simulink model "AirRefueling_Platform_Varyingmass"  (R2023a)
settings: Solver=VariableStepAuto  StartTime=0.0  StopTime=100  FixedStep=0.01  RelTol=1e-3  EnableMultiTasking=on
InitFcn:
  | F16_Init
values from neighbouring files (symbols this model uses):
  A_define = A(1:12,1:12)    [F16_Init.m]
  airSpeed = 393.72    [F16_Init.m]
  alpha0 = trimAlpha*180/pi    (= 6.62393794015)    [F16_Init.m]
  altitude = 9843    [F16_Init.m]
  B_define = A(1:12,13:16)    [F16_Init.m]
  b_ref = 30.0    (= 30)    [F16_Init.m]
  C = [ 1,0,0,zeros(1,15) ... (first row only)    [F16_Init.m]
  C2m = [C(1,:) ... (first row only)    [F16_Init.m]
  C_la = [1,0,zeros(1,4)]    [F16_Init.m]
  C_lon = [1,0,zeros(1,4);0,1,zeros(1,4)]    [F16_Init.m]
  Cdr_ = 0.8    [HoseDrogue_Parameter.m]
  d_f_rc = [3.75;0;-1.75]    [F16_Init.m]
  d_pr_cam = d_pr_rc - d_cam_rc    [F16_Init.m]
  d_pr_rc = [7.6;0.50;-2.44]    [F16_Init.m]
  dLEF = 0    [F16_Init.m]
  dtheta10 = zeros(1,N)    [HoseDrogue_Parameter.m]
  dtheta20 = zeros(1,N)    [HoseDrogue_Parameter.m]
  fi_flag = 1    [F16_Init.m]
  height = 3000    [HoseDrogue_Parameter.m]
  Inertia = [9496,0,-982.0;0,55814.0,0;-982.0,0,63100.0]    [F16_Init.m]
  k_reel = 0.5    [HoseDrogue_Parameter.m]
  Kc = [ ... (first row only)    [F16_Init.m]
  kd = 500    [HoseDrogue_Parameter.m]
  Ki = zeros(4,3)    [F16_Init.m]
  Ki_la = -k_la(:,9)    [F16_Init.m]
  Ki_lon = -k_lon(:,9:10)    [F16_Init.m]
  Kp = zeros(4,18)    [F16_Init.m]
  kp_la = Kp_define(3:4,[2,4,6,9,10,12])    [F16_Init.m]
  kp_lon = Kp_define(1:2,[1,3,5,7,8,11])    [F16_Init.m]
  l0 = (length-l1)/(N-1)    (= 1.44444444444)    [HoseDrogue_Parameter.m]
  l1 = 2    [HoseDrogue_Parameter.m]
  l_density = 4.1    [HoseDrogue_Parameter.m]
  m0 = l0*l_density    (= 5.92222222222)    [HoseDrogue_Parameter.m]
  mass = 636.94    [F16_Init.m]
  Mdr = 29.5    [HoseDrogue_Parameter.m]
  N = 10    [HoseDrogue_Parameter.m]    (also in bsp3.m)
  p0_rc = [-30;1;8]    [F16_Init.m]
  Rdr = 0.305    [HoseDrogue_Parameter.m]
  Rl = 0.0336    [HoseDrogue_Parameter.m]
  T_reel_initial = 1610    [HoseDrogue_Parameter.m]
  theta10 = theta1_100    [HoseDrogue_Parameter.m]
  theta20 = theta2_100    [HoseDrogue_Parameter.m]
  trim_ail = 0.00874607850103852    (= 0.00874607850104)    [F16_Init.m]
  trim_control = [trim_thrust;trim_ele;trim_ail;trim_rud]    [F16_Init.m]
  trim_ele = -2.97973164860638    (= -2.97973164861)    [F16_Init.m]
  trim_rud = 0.0680302158182712    (= 0.0680302158183)    [F16_Init.m]
  trim_state = [0;0;0;0;trimAlpha;0;airSpeed;trimAlpha;0;0;0;0]    [F16_Init.m]
  trim_state1 = [trim_state;0;0;0;0;0;0]    [F16_Init.m]
  trim_thrust = 2279.08519954656    (= 2279.08519955)    [F16_Init.m]
  visual_err = [0.07;0.04;-1.21]    [F16_Init.m]
  vt0 = [120;0;0]    [HoseDrogue_Parameter.m]
undefined symbols (not defined in the file or in its folder): A_la_define, A_lon_define, B_la_define, B_lon_define, CC_la, CC_lon, dockingPoint, F, Light, MIL, STD, v_oil
libraries: aerolibconvert2 x13, etargetslib x11, dspnetwork x10, aerolibasang x8, aerolibatmos2 x3, aerolibobsolete x3, simulink x2, aerolibwind2 x2, aerolibadyn x2, sharedtransform x2, aerolibutil x2, vrlib x1
(part 2 of 4)

== system AirRefueling_Platform_Varyingmass/Receiver system/Controller ==
  note: u
  note: -kx
  note: u'
  note: e
  note: 跟踪控制
      | 设计反馈矩阵 Ki 使得误差 e 收敛为0
  note: x'=Ax+Bu
      | 增稳控制 u = Kp * x
      | 设计反馈矩阵 Kp 配置极点
  Ori_states : Inport
  C : Gain  Commented=on  Gain=C  Multiplication=Matrix(K*u) (u vector)
  Constant : Constant  Commented=on  Value=trim_control
  Demux : Demux  Commented=on
  Demux1 : Demux  Commented=on  Outputs=3
  Display : Display  Commented=on
  Gain : Gain  Commented=on  Gain=1000
  Gain1 : Gain  Commented=on  Gain=[1,0,0;0,0,-1;0,1,0]  Multiplication=Matrix(K*u) (u vector)
  Integrator : Integrator  Commented=on
  Integrator1 : Integrator  Commented=on
  Integrator2 : Integrator  Commented=on
  Ki : Gain  Commented=on  Gain=Ki  Multiplication=Matrix(K*u) (u vector)
  Kp : Gain  Commented=on  Gain=Kp  Multiplication=Matrix(K*u) (u vector)
  Length Conversion : aerolibconvert2/Length Conversion  Commented=on  IU=m  OU=ft
  Mux : Mux  Commented=on
  Mux3 : Mux  Commented=on  Inputs=3
  Observer1 : Subsystem
  Saturation : Saturate  Commented=on  UpperLimit=15  LowerLimit=-15
  Sum : Sum  Commented=on  Inputs=|++
  Sum2 : Sum  Commented=on  Inputs=|+-
  Sum3 : Sum  Commented=on  Inputs=+|-
  Sum4 : Sum  Inputs=|++
  pri_sys_controller1 : Subsystem
  sec_sys_controller1 : Subsystem
  Out1 : Outport
  wires:
  Sum2/1 -> Demux1/1
  C/1 -> Sum2/2
  Mux3/1 -> Ki/1
  Demux1/2 -> Integrator1/1
  Integrator1/1 -> Mux3/2
  Integrator/1 -> Mux3/1
  Demux1/3 -> Integrator2/1
  Integrator2/1 -> Mux3/3
  Length Conversion/1 -> Sum2/1
  Demux1/1 -> Saturation/1
  Ki/1 -> Sum3/1
  Kp/1 -> Sum3/2
  Sum3/1 -> Demux/1
  Saturation/1 -> Integrator/1
  Demux/2 -> Mux/2
  Demux/3 -> Mux/3
  Demux/4 -> Mux/4
  Demux/1 -> Gain/1
  Gain/1 -> Mux/1
  ? -> Gain1/1
  Gain1/1 -> Length Conversion/1
  Constant/1 -> Sum/2
  Mux/1 -> Sum/1
  sec_sys_controller1/1(Sec_inputs) -> Observer1/1(Sec_input), Sum4/2
  Ori_states/1 -> Observer1/2(Ori_states)
  Sum4/1 -> Out1/1
  Observer1/1(Sec_Obv_States) -> sec_sys_controller1/2(Sec_Obv_States)
  Observer1/2(Pri_Obv_States) -> sec_sys_controller1/1(Pri_Obv_States), pri_sys_controller1/1(Pri_Obv_States)
  pri_sys_controller1/1(Pri_inputs) -> Sum4/1

== system AirRefueling_Platform_Varyingmass/Receiver system/F16 Nonlinear Model ==
  u2 : Inport
  u4 : Inport  Port=2
  Variable Mass Model : Subsystem
  constant mass model : Subsystem
  state2 : Outport
  Out2 : Outport  Port=2
  state3 : Outport  Port=3
  wires:
  u4/1 -> Variable Mass Model/1(u4)
  Variable Mass Model/1(state2) -> state2/1
  Variable Mass Model/2(Out2) -> Out2/1
  Variable Mass Model/3(state3) -> state3/1
  u2/1 -> constant mass model/1(u2)
  constant mass model/1(V_wind) -> Variable Mass Model/2(Wind Velocity)
  constant mass model/2(W_wind) -> Variable Mass Model/3(Wind Angular Rates)

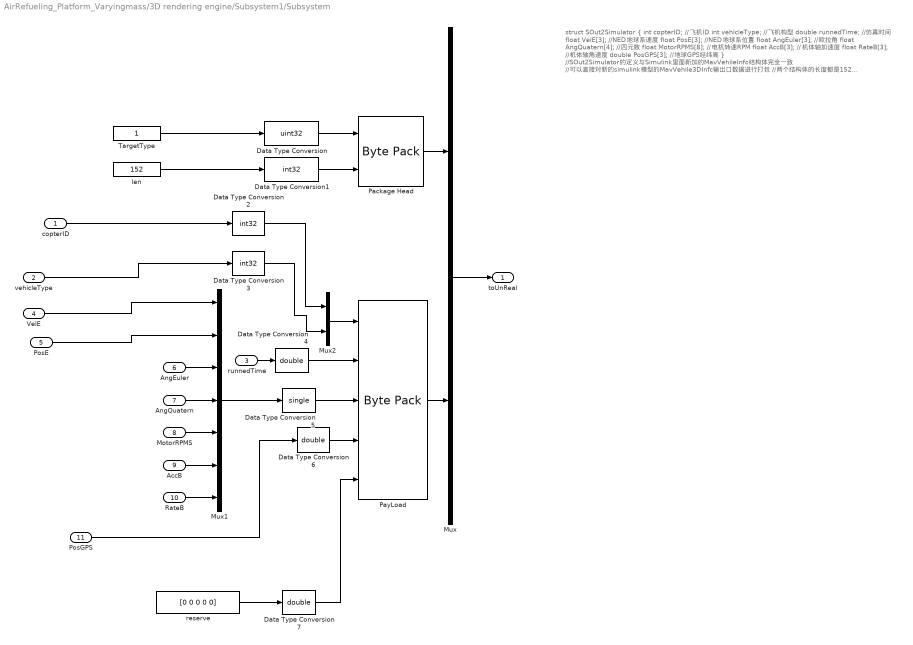
== system AirRefueling_Platform_Varyingmass/3D rendering engine/Subsystem1/Subsystem ==
  note: struct SOut2Simulator
      | {
      | int copterID; //飞机ID
      | int vehicleType; //飞机构型
      | double runnedTime; //仿真时间
      | float VelE[3]; //NED地球系速度
      | float PosE[3]; //NED地球系位置
      | float AngEuler[3]; //欧拉角
      | float AngQuatern[4]; //四元数
      | float MotorRPMS[8]; //电机转速RPM
      | float AccB[3]; //机体轴加速度
      | float RateB[3]; //机体轴角速度
      | double PosGPS[3]; //地球GPS经纬高
      | }
      |
      | //SOut2Simulator的定义与Simulink里面新加的MavVehileInfo结构体完全一致
      | //可以直接对新的simulink模型的MavVehile3DInfo输出口数据进行打包
      | //两个结构体的长度都是152
      | sizeof(SOut2Simulator) = sizeof(MavVehileInfo) = 152
      |
      | 打包封装的结构体为
      | typedef struct _netDataShort
      | {
      | TargetType tg; //这里目前随便填，写1即可 uint32
      | int len; //这个长度为传输结构体长度，目前是152
      | char payload[192]; //这里面前152位存放了SOut2Simulator结构体数据，后面的40位保留
      | }netDataShort;
      |
      | //UDP包的总长度为200
      | sizeof(netDataShort) = 200
      |
      | //发送的UDP端口号为：20010
  copterID : Inport  PortDimensions=1
  vehicleType : Inport  Port=2  PortDimensions=1
  runnedTime : Inport  Port=3  PortDimensions=1
  "VelE " : Inport  Port=4  PortDimensions=3
  PosE : Inport  Port=5  PortDimensions=3
  AngEuler : Inport  Port=6  PortDimensions=3
  AngQuatern : Inport  Port=7  PortDimensions=4
  MotorRPMS : Inport  Port=8  PortDimensions=8
  AccB : Inport  Port=9  PortDimensions=3
  RateB : Inport  Port=10  PortDimensions=3
  PosGPS : Inport  Port=11  PortDimensions=3
  Data Type Conversion : DataTypeConversion  OutDataTypeStr=uint32  SaturateOnIntegerOverflow=off  RndMeth=Floor
  Data Type Conversion1 : DataTypeConversion  OutDataTypeStr=int32  SaturateOnIntegerOverflow=off  RndMeth=Floor
  Data Type Conversion2 : DataTypeConversion  OutDataTypeStr=int32  SaturateOnIntegerOverflow=off  RndMeth=Floor
  Data Type Conversion3 : DataTypeConversion  OutDataTypeStr=int32  SaturateOnIntegerOverflow=off  RndMeth=Floor
  Data Type Conversion4 : DataTypeConversion  OutDataTypeStr=double  SaturateOnIntegerOverflow=off  RndMeth=Floor
  Data Type Conversion5 : DataTypeConversion  OutDataTypeStr=single  SaturateOnIntegerOverflow=off  RndMeth=Floor
  Data Type Conversion6 : DataTypeConversion  OutDataTypeStr=double  SaturateOnIntegerOverflow=off  RndMeth=Floor
  Data Type Conversion7 : DataTypeConversion  OutDataTypeStr=double  SaturateOnIntegerOverflow=off  RndMeth=Floor
  Mux : Mux  Inputs=2
  Mux1 : Mux  Inputs=7
  Mux2 : Mux  Inputs=2
  Package Head : etargetslib/Byte Pack  datatypes={'uint32','int32'}  byteAlign=4
  PayLoad : etargetslib/Byte Pack  datatypes={'int32','double','single','double','double'}  byteAlign=8
  TargetType : Constant  OutDataTypeStr=Inherit: Inherit via back propagation
  len : Constant  Value=152  OutDataTypeStr=Inherit: Inherit via back propagation
  reserve : Constant  Value=[0 0 0 0 0]  OutDataTypeStr=double
  toUnReal : Outport  VectorParamsAs1DForOutWhenUnconnected=off
  wires:
  runnedTime/1 -> Data Type Conversion4/1
  RateB/1 -> Mux1/7
  PayLoad/1 -> Mux/2
  "VelE "/1 -> Mux1/1
  Mux1/1 -> Data Type Conversion5/1
  PosGPS/1 -> Data Type Conversion6/1
  Package Head/1 -> Mux/1
  AccB/1 -> Mux1/6
  Mux/1 -> toUnReal/1
  MotorRPMS/1 -> Mux1/5
  AngQuatern/1 -> Mux1/4
  copterID/1 -> Data Type Conversion2/1
  len/1 -> Data Type Conversion1/1
  vehicleType/1 -> Data Type Conversion3/1
  PosE/1 -> Mux1/2
  TargetType/1 -> Data Type Conversion/1
  reserve/1 -> Data Type Conversion7/1
  Mux2/1 -> PayLoad/1
  AngEuler/1 -> Mux1/3
  Data Type Conversion5/1 -> PayLoad/3
  Data Type Conversion2/1 -> Mux2/1
  Data Type Conversion1/1 -> Package Head/2
  Data Type Conversion6/1 -> PayLoad/4
  Data Type Conversion/1 -> Package Head/1
  Data Type Conversion3/1 -> Mux2/2
  Data Type Conversion4/1 -> PayLoad/2
  Data Type Conversion7/1 -> PayLoad/5

== system AirRefueling_Platform_Varyingmass/Hose-drogue system/DRdynamics/HDU ==
  note: 第一根管子的a
  t_hose : Inport
  Compare To Zero : simulink/Logic and Bit Operations/Compare To Zero  Commented=on  relop=<=  OutDataTypeStr=boolean
  Divide : Product  Inputs=*/
  Integrator : Integrator  ExternalReset=rising  UpperSaturationLimit=0.3  LowerSaturationLimit=-0.3
  Integrator1 : Integrator  ExternalReset=rising  InitialCondition=l1
  MATLAB Function1 : MATLAB Function  TreatAsAtomicUnit=on
  MATLAB Function2 : MATLAB Function  TreatAsAtomicUnit=on
  Memory2 : Memory  InitialCondition=l1
  Memory3 : Memory
  Saturation : Saturate  UpperLimit=3  LowerLimit=-3
  Scope{1..3,5,7..8} (6 alike) : Scope
  Stop Simulation : Stop  Commented=on
  To Workspace3 : ToWorkspace  VariableName=l1  SampleTime=-1
  l1 initial1 : Constant  Value=l1
  m_reel : Constant  Value=68
  t_reel : Constant  Value=T_reel_initial
  l_1 : Outport
  dl_1 : Outport  Port=2
  ddl_1 : Outport  Port=3
  wires:
  MATLAB Function2/1(Tt) -> Scope3/1, Divide/1
  m_reel/1 -> Divide/2
  Divide/1 -> Saturation/1, Scope2/1  "ddl_1"
  Integrator/1 -> Integrator1/1, MATLAB Function1/3(dl1), MATLAB Function2/4(dl), Scope8/1  "dl_k"
  Saturation/1 -> MATLAB Function1/4(ddl1), Integrator/1, Scope5/1
  t_reel/1 -> MATLAB Function2/2(T0)
  Compare To Zero/1 -> Stop Simulation/1
  l1 initial1/1 -> MATLAB Function1/2(l1initial)
  MATLAB Function1/4(ddl1out) -> Scope7/1, ddl_1/1
  MATLAB Function1/1(flag1) -> Memory3/1
  Memory2/1 -> MATLAB Function2/1(l_1)
  Memory3/1 -> Integrator/2, Integrator1/2
  Integrator1/1 -> MATLAB Function1/1(l1), Compare To Zero/1, To Workspace3/1, Memory2/1, Scope1/1
  MATLAB Function1/2(l1out) -> l_1/1
  MATLAB Function1/3(dl1out) -> dl_1/1
  t_hose/1 -> MATLAB Function2/3(t)

== system AirRefueling_Platform_Varyingmass/Hose-drogue system/DRdynamics/Hose-Drogue1 ==
  note: % vr = 连杆相对风速度 向量3*N
      | % n = 连杆的方向向量，向上为正 向量3*N
  note: link1的加速度
  note: tanker的加速度
  note: 3*N的数组
  note: 扰动等的力
  note: 高度生成密度和粘滞系数
  pt : Inport
  vt : Inport  Port=2
  at : Inport  Port=3
  w : Inport  Port=4
  link length : Inport  Port=5
  D link length : Inport  Port=6
  DD link length : Inport  Port=7
  Fb : Inport  Port=8
  Atmosphere Data : Subsystem
  Calculate the Acceleration of the Links1 : Subsystem
  Calculate the External Force of the Links : Subsystem
  Calculate the Orientation of the Links1 : Subsystem
  Height : Constant  Value=height
  MATLAB Function3 : MATLAB Function  TreatAsAtomicUnit=on
  Scope : Scope
  Scope1 : Scope
  Scope8 : Scope
  link line density : Constant  Value=l_density
  link radius : Constant  Value=Rl
  p link : Outport
  t : Outport  Port=2
  pdr : Outport  Port=3
  wires:
  Height/1 -> Atmosphere Data/1(height)
  Atmosphere Data/1(densitiy) -> Calculate the External Force of the Links/6(density)
  Atmosphere Data/2(viscosity) -> Calculate the External Force of the Links/7(viscosity)
  link radius/1 -> Calculate the External Force of the Links/4(link radius)
  link line density/1 -> Calculate the External Force of the Links/5(link line density), Calculate the Acceleration of the Links1/5(link line density)
  Calculate the External Force of the Links/1(Q) -> Scope/1, Calculate the Acceleration of the Links1/1(Q)
  Calculate the Orientation of the Links1/1(n) -> Calculate the External Force of the Links/2(n), MATLAB Function3/1(n), Calculate the Acceleration of the Links1/3(n)
  Calculate the Orientation of the Links1/2(dn) -> Calculate the Acceleration of the Links1/4(dn)
  Calculate the External Force of the Links/2(Mdr) -> Calculate the Acceleration of the Links1/2(Mdr)
  at/1 -> Calculate the Orientation of the Links1/4(at), Calculate the Acceleration of the Links1/8("tanker acceleration ")
  Calculate the Orientation of the Links1/3(vr) -> Calculate the External Force of the Links/1(vr)
  w/1 -> Calculate the Orientation of the Links1/6(w)
  Calculate the Acceleration of the Links1/1(a) -> Calculate the Orientation of the Links1/3(a), Scope8/1
  Calculate the Orientation of the Links1/4(p) -> Calculate the External Force of the Links/8(p), p link/1
  pt/1 -> Calculate the Orientation of the Links1/7(pt)
  vt/1 -> Calculate the Orientation of the Links1/5(vt)
  Calculate the Acceleration of the Links1/2(t) -> t/1
  link length/1 -> Calculate the Orientation of the Links1/1(link length), Calculate the External Force of the Links/3(l1), Calculate the Acceleration of the Links1/6(l1 length)
  D link length/1 -> Calculate the Orientation of the Links1/2(D link length)
  DD link length/1 -> Calculate the Acceleration of the Links1/7(DD l1 length)
  Fb/1 -> Calculate the External Force of the Links/9(Fb)
  MATLAB Function3/1(alpha) -> Scope1/1
  Calculate the Orientation of the Links1/5(pdr) -> pdr/1

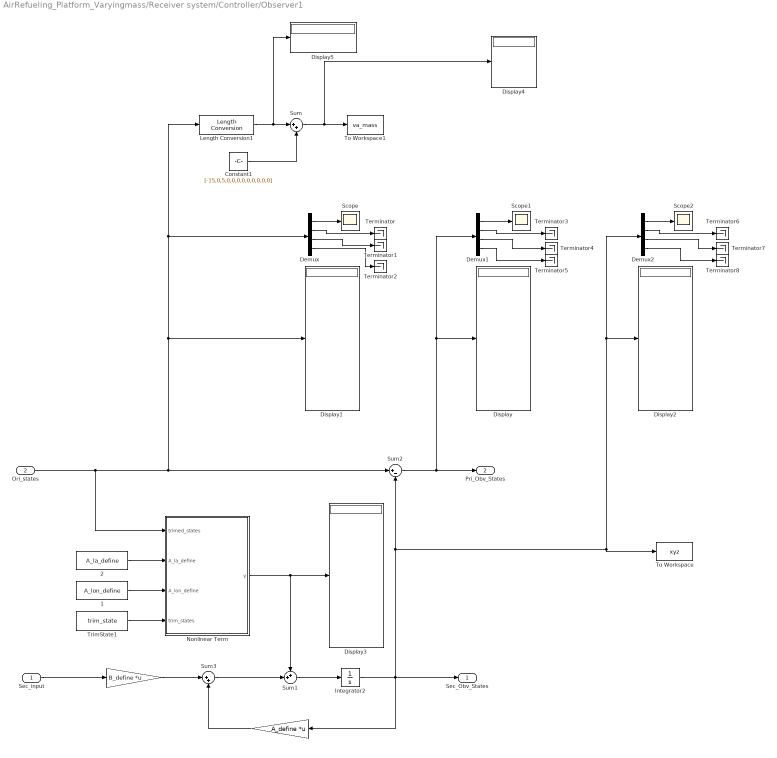
== system AirRefueling_Platform_Varyingmass/Receiver system/Controller/Observer1 ==
  Sec_input : Inport
  Ori_states : Inport  Port=2
  " " : Gain  Gain=A_define  Multiplication=Matrix(K*u) (u vector)
  "  " : Gain  Gain=B_define  Multiplication=Matrix(K*u) (u vector)
  " 1" : Constant  Value=A_lon_define
  " 2" : Constant  Value=A_la_define
  Constant1 : Constant  Value=[-15,0,5,0,0,0,0,0,0,0,0,0]
  Demux : Demux
  Demux1 : Demux
  Demux2 : Demux
  Display{,1..5} (6 alike) : Display
  Integrator2 : Integrator
  Length Conversion1 : aerolibconvert2/Length Conversion  IU=ft  OU=m
  Nonlinear Term : MATLAB Function  TreatAsAtomicUnit=on
  Scope : Scope
  Scope1 : Scope
  Scope2 : Scope
  Sum : Sum  Inputs=|++
  Sum1 : Sum  Inputs=++|
  Sum2 : Sum  Inputs=|+-
  Sum3 : Sum  Inputs=|++
  Terminator{,1..8} (9 alike) : Terminator
  To Workspace : ToWorkspace  VariableName=xyz  SaveFormat=Structure With Time  SampleTime=1
  To Workspace1 : ToWorkspace  VariableName=va_mass  SaveFormat=Structure With Time  SampleTime=-1
  TrimState1 : Constant  Value=trim_state
  Sec_Obv_States : Outport  VectorParamsAs1DForOutWhenUnconnected=off
  Pri_Obv_States : Outport  Port=2  VectorParamsAs1DForOutWhenUnconnected=off
  wires:
  Sec_input/1 -> "  "/1
  "  "/1 -> Sum3/1
  " "/1 -> Sum3/2
  Sum3/1 -> Sum1/2
  Sum1/1 -> Integrator2/1
  Integrator2/1 -> Sec_Obv_States/1, " "/1, Demux2/1, Display2/1, To Workspace/1, Sum2/2
  Sum2/1 -> Display/1, Demux1/1, Pri_Obv_States/1
  " 1"/1 -> Nonlinear Term/3(A_lon_define)
  " 2"/1 -> Nonlinear Term/2(A_la_define)
  Demux/1 -> Scope/1
  Demux1/1 -> Scope1/1
  Demux2/1 -> Scope2/1
  Nonlinear Term/1(y) -> Display3/1, Sum1/1
  Ori_states/1 -> Nonlinear Term/1(trimed_states), Sum2/1, Display1/1, Length Conversion1/1, Demux/1
  TrimState1/1 -> Nonlinear Term/4(trim_states)
  Length Conversion1/1 -> Display5/1, Sum/1
  Constant1/1 -> Sum/2
  Demux/2 -> Terminator/1
  Demux/4 -> Terminator2/1
  Demux/3 -> Terminator1/1
  Demux1/2 -> Terminator3/1
  Demux1/3 -> Terminator4/1
  Demux1/4 -> Terminator5/1
  Demux2/2 -> Terminator6/1
  Demux2/4 -> Terminator8/1
  Demux2/3 -> Terminator7/1
  Sum/1 -> Display4/1, To Workspace1/1

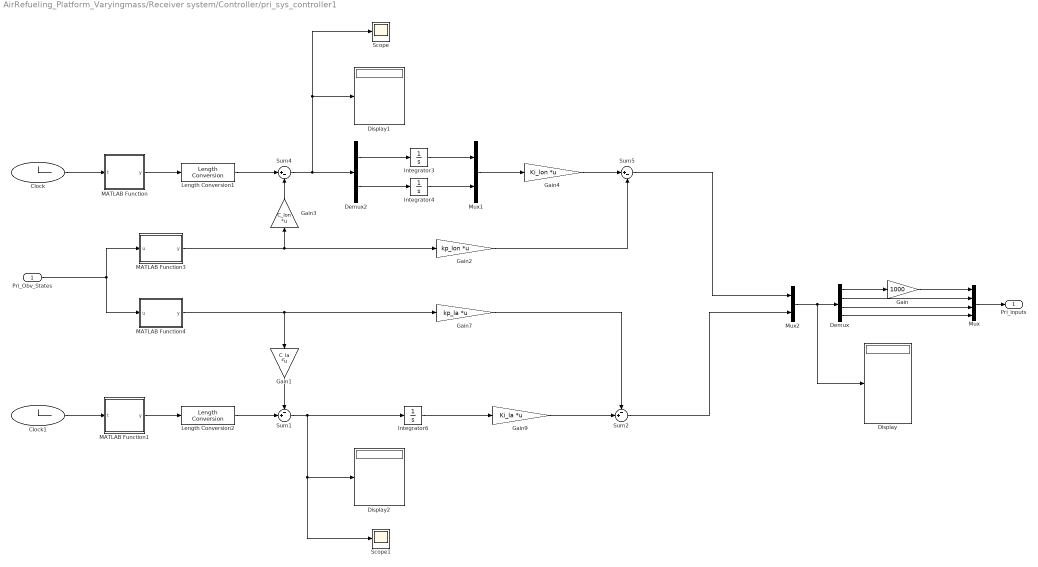
== system AirRefueling_Platform_Varyingmass/Receiver system/Controller/pri_sys_controller1 ==
  Pri_Obv_States : Inport
  Clock : Clock
      settings: Decimation=50
  Clock1 : Clock
      settings: Decimation=50
  Demux : Demux
  Demux2 : Demux  Outputs=2
  Display : Display
  Display1 : Display
  Display2 : Display
  Gain : Gain  Gain=1000
  Gain1 : Gain  Gain=C_la  Multiplication=Matrix(K*u) (u vector)
  Gain2 : Gain  Gain=kp_lon  Multiplication=Matrix(K*u) (u vector)
  Gain3 : Gain  Gain=C_lon  Multiplication=Matrix(K*u) (u vector)
  Gain4 : Gain  Gain=Ki_lon  Multiplication=Matrix(K*u) (u vector)
  Gain7 : Gain  Gain=kp_la  Multiplication=Matrix(K*u) (u vector)
  Gain9 : Gain  Gain=Ki_la  Multiplication=Matrix(K*u) (u vector)
  Integrator3 : Integrator
  Integrator4 : Integrator
  Integrator6 : Integrator
  Length Conversion1 : aerolibconvert2/Length Conversion  IU=m  OU=ft
  Length Conversion2 : aerolibconvert2/Length Conversion  IU=m  OU=ft
  MATLAB Function : MATLAB Function  TreatAsAtomicUnit=on
  MATLAB Function1 : MATLAB Function  TreatAsAtomicUnit=on
  MATLAB Function3 : MATLAB Function  TreatAsAtomicUnit=on
  MATLAB Function4 : MATLAB Function  TreatAsAtomicUnit=on
  Mux : Mux
  Mux1 : Mux  Inputs=2
  Mux2 : Mux  Inputs=2
  Scope : Scope
  Scope1 : Scope
  Sum1 : Sum  Inputs=-+|
  Sum2 : Sum  Inputs=-+|
  Sum4 : Sum  Inputs=|+-
  Sum5 : Sum  Inputs=|+-
  Pri_inputs : Outport  VectorParamsAs1DForOutWhenUnconnected=off
  wires:
  Pri_Obv_States/1 -> MATLAB Function3/1(u), MATLAB Function4/1(u)
  Gain2/1 -> Sum5/2
  MATLAB Function/1(y) -> Length Conversion1/1
  Sum4/1 -> Display1/1, Scope/1, Demux2/1
  Demux2/2 -> Integrator4/1
  Integrator4/1 -> Mux1/2
  Integrator3/1 -> Mux1/1
  Mux1/1 -> Gain4/1
  Gain3/1 -> Sum4/2
  Gain4/1 -> Sum5/1
  Clock/1 -> MATLAB Function/1(t)
  Length Conversion1/1 -> Sum4/1
  Demux/2 -> Mux/2
  Demux/3 -> Mux/3
  Demux/4 -> Mux/4
  Demux/1 -> Gain/1
  Gain/1 -> Mux/1
  Mux/1 -> Pri_inputs/1
  MATLAB Function1/1(y) -> Length Conversion2/1
  Sum1/1 -> Display2/1, Scope1/1, Integrator6/1
  Integrator6/1 -> Gain9/1
  Clock1/1 -> MATLAB Function1/1(t)
  MATLAB Function3/1(y) -> Gain2/1, Gain3/1
  MATLAB Function4/1(y) -> Gain7/1, Gain1/1
  Length Conversion2/1 -> Sum1/2
  Gain1/1 -> Sum1/1
  Gain9/1 -> Sum2/2
  Gain7/1 -> Sum2/1
  Sum5/1 -> Mux2/1
  Sum2/1 -> Mux2/2
  Demux2/1 -> Integrator3/1
  Mux2/1 -> Display/1, Demux/1

== system AirRefueling_Platform_Varyingmass/Receiver system/Controller/sec_sys_controller1 ==
  Pri_Obv_States : Inport
  Sec_Obv_States : Inport  Port=2
  " " : Constant  Value=A_lon_define
  "    " : Constant  Value=B_lon_define
  "     " : Constant  Value=A_la_define
  "      " : Constant  Value=B_la_define
  "    1" : Constant  Value=CC_lon
  "    2" : Constant  Value=CC_la
  Demux : Demux
  Gain1 : Gain  Gain=1000
  Lat_Controller : MATLAB Function  TreatAsAtomicUnit=on
  Lon_Controller : MATLAB Function  TreatAsAtomicUnit=on
  Mux : Mux
  Mux13 : Mux  Inputs=2
  Scope : Scope
  Scope1 : Scope
  TrimState1 : Constant  Value=trim_state
  TrimState2 : Constant  Value=trim_state
  Sec_inputs : Outport  VectorParamsAs1DForOutWhenUnconnected=off
  wires:
  Demux/1 -> Gain1/1
  Gain1/1 -> Mux/1
  Mux/1 -> Sec_inputs/1
  Demux/2 -> Mux/2
  Demux/3 -> Mux/3
  Demux/4 -> Mux/4
  Lon_Controller/2(output) -> Mux13/1
  " "/1 -> Lon_Controller/3(A_lon_define)
  "    "/1 -> Lon_Controller/4(B_lon_define)
  "     "/1 -> Lat_Controller/3(A_la_define)
  "      "/1 -> Lat_Controller/4(B_la_define)
  Lat_Controller/1(output) -> Mux13/2
  "    1"/1 -> Lon_Controller/5(CC_lon)
  "    2"/1 -> Lat_Controller/5(CC_la)
  Lon_Controller/1(s) -> Scope/1
  Lat_Controller/2(s) -> Scope1/1
  Mux13/1 -> Demux/1
  Sec_Obv_States/1 -> Lat_Controller/2(Sec_States), Lon_Controller/1(Sec_States)
  Pri_Obv_States/1 -> Lat_Controller/1(Pri_States), Lon_Controller/2(Pri_States)
  TrimState1/1 -> Lat_Controller/6(trim_states)
  TrimState2/1 -> Lon_Controller/6(trim_states)

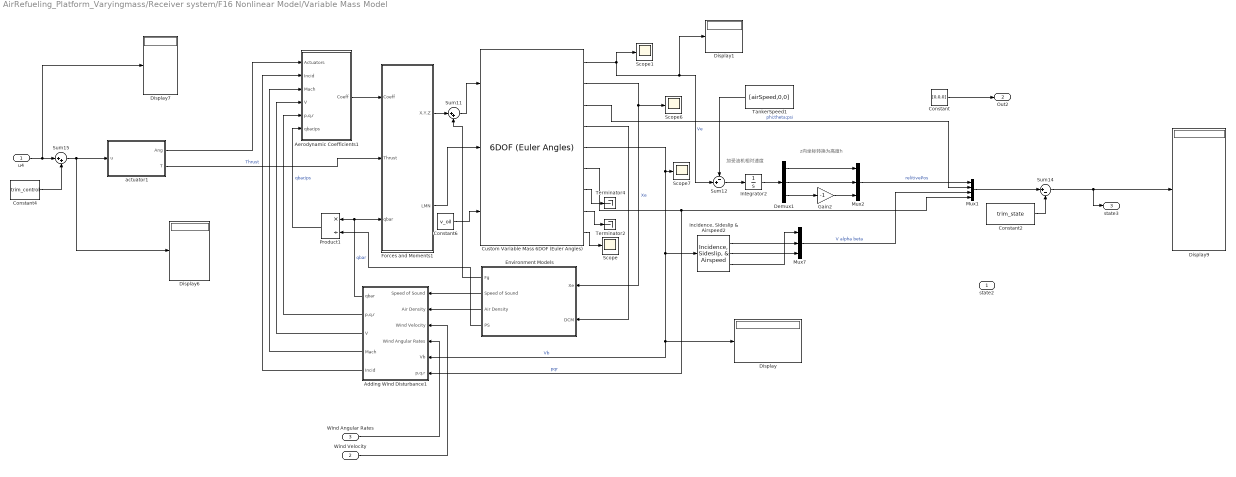
== system AirRefueling_Platform_Varyingmass/Receiver system/F16 Nonlinear Model/Variable Mass Model ==
  note: z向坐标转换为高度h
  note: 加受油机相对速度
  u4 : Inport
  Wind Velocity : Inport  Port=2
  Wind Angular Rates : Inport  Port=3
  Adding Wind Disturbance1 : Subsystem
  Aerodynamic Coefficients1 : Subsystem
  Constant : Constant  Value=[0,0,0]
  Constant2 : Constant  Value=trim_state
  Constant4 : Constant  Value=trim_control
  Constant6 : Constant  Value=v_oil
  Custom Variable Mass 6DOF (Euler Angles) : shared6dof/6DOF (Euler Angles)  units=English (Velocity in ft/s)  mtype=Simple Variable  rep=Euler Angles  xme_0=xyz_0  Vm_0=uvw_0  eul_0=Euler_0  pm_0=pqr  mass_0=1.0*mass  mass_e=1.0*mass  mass_f=1.0*mass + 137  inertia=eye(3)  inertia_e=Inertia  inertia_f=1.37*Inertia  k_quat=1.0  vre_flag=off  abi_flag=off  aMode=aMode  xme_statename=''  Vm_statename=''  eul_statename=''  quat_statename=''  pm_statename=''  mass_statename=''
  Demux1 : Demux  Outputs=3
  Display{,1,6..7,9} (5 alike) : Display
  Environment Models : Subsystem
  Forces and Moments1 : Subsystem
  Gain2 : Gain  Gain=-1
  "Incidence, Sideslip & Airspeed2" : aerolibasang/Incidence, Sideslip, & Airspeed
  Integrator2 : Integrator
  Mux1 : Mux
  Mux2 : Mux  Inputs=3
  Mux7 : Mux  Inputs=3
  Product1 : Product  Inputs=*/  InputSameDT=on  SaturateOnIntegerOverflow=on  OutDataTypeStr=Inherit: Same as first input
  Scope{,1,6..7} (4 alike) : Scope
  Sum11 : Sum  Inputs=|++  InputSameDT=on  SaturateOnIntegerOverflow=on  OutDataTypeStr=Inherit: Same as first input
  Sum12 : Sum  Inputs=-+|
  Sum14 : Sum  Inputs=|+-
  Sum15 : Sum  Inputs=|++
  TankerSpeed1 : Constant  Value=[airSpeed,0,0]
  Terminator2 : Terminator
  Terminator4 : Terminator
  actuator1 : Subsystem
  state2 : Outport
  Out2 : Outport  Port=2
  state3 : Outport  Port=3
  wires:
  Adding Wind Disturbance1/1(qbar) -> Forces and Moments1/3(qbar), Product1/1  "qbar"
  Mux1/1 -> Sum14/1
  Sum15/1 -> Display6/1, actuator1/1(u)
  Custom Variable Mass 6DOF (Euler Angles)/6 -> Mux1/4, Adding Wind Disturbance1/6(p,q,r)  "pqr"
  Sum14/1 -> Display9/1, state3/1
  Custom Variable Mass 6DOF (Euler Angles)/3 -> Mux1/2  "phi;theta;psi"
  Gain2/1 -> Mux2/3
  u4/1 -> Display7/1, Sum15/1
  Wind Angular Rates/1 -> Adding Wind Disturbance1/4(Wind Angular Rates)
  "Incidence, Sideslip & Airspeed2"/2 -> Mux7/3
  Custom Variable Mass 6DOF (Euler Angles)/4 -> Environment Models/2(DCM)
  Constant2/1 -> Sum14/2
  TankerSpeed1/1 -> Sum12/1
  actuator1/1(Ang) -> Aerodynamic Coefficients1/1(Actuators)
  "Incidence, Sideslip & Airspeed2"/3 -> Mux7/1
  Adding Wind Disturbance1/4(Mach) -> Aerodynamic Coefficients1/3(Mach)
  Environment Models/1(Fg) -> Sum11/2
  Custom Variable Mass 6DOF (Euler Angles)/1 -> Display1/1, Sum12/2, Scope1/1  "Ve"
  Demux1/3 -> Gain2/1
  Custom Variable Mass 6DOF (Euler Angles)/8 -> Terminator2/1
  Adding Wind Disturbance1/2("p,q,r ") -> Aerodynamic Coefficients1/5(p,q,r)
  Forces and Moments1/1(X,Y,Z) -> Sum11/1
  actuator1/2(T) -> Forces and Moments1/2(Thrust)  "Thrust"
  Adding Wind Disturbance1/3(V) -> Aerodynamic Coefficients1/4(V)
  Product1/1 -> Aerodynamic Coefficients1/6(qbar/ps)  "qbar/ps"
  Sum12/1 -> Integrator2/1
  Demux1/2 -> Mux2/2
  Custom Variable Mass 6DOF (Euler Angles)/5 -> Scope7/1, Display/1, Adding Wind Disturbance1/5(Vb), "Incidence, Sideslip & Airspeed2"/1  "Vb"
  Aerodynamic Coefficients1/1(Coeff) -> Forces and Moments1/1(Coeff)
  Custom Variable Mass 6DOF (Euler Angles)/7 -> Terminator4/1
  Constant6/1 -> Custom Variable Mass 6DOF (Euler Angles)/3
  Forces and Moments1/2(LMN) -> Custom Variable Mass 6DOF (Euler Angles)/2
  Constant4/1 -> Sum15/2
  Environment Models/2(Speed of Sound) -> Adding Wind Disturbance1/1(Speed of Sound)
  Integrator2/1 -> Demux1/1
  Environment Models/4(PS) -> Product1/2
  Custom Variable Mass 6DOF (Euler Angles)/2 -> Environment Models/1(Xe), Scope6/1  "Xe"
  Demux1/1 -> Mux2/1
  Adding Wind Disturbance1/5(Incid) -> Aerodynamic Coefficients1/2(Incid)
  Environment Models/3(Air Density) -> Adding Wind Disturbance1/2(Air Density)
  Custom Variable Mass 6DOF (Euler Angles)/9 -> Scope/1
  "Incidence, Sideslip & Airspeed2"/1 -> Mux7/2
  Sum11/1 -> Custom Variable Mass 6DOF (Euler Angles)/1
  Wind Velocity/1 -> Adding Wind Disturbance1/3(Wind Velocity)
  Mux2/1 -> Mux1/1  "relitivePos"
  Mux7/1 -> Mux1/3  "V alpha beta"
  Constant/1 -> Out2/1

== system AirRefueling_Platform_Varyingmass/Receiver system/F16 Nonlinear Model/constant mass model ==
  note: Up
  note: Us
  u2 : Inport
  F-16 : Subsystem
  Observer : Subsystem
  Sum1 : Sum  Inputs=|++
  pri_sys_controller : Subsystem
  sec_sys_controller : Subsystem
  V_wind : Outport
  W_wind : Outport  Port=2
  wires:
  F-16/1(state1) -> Observer/2(Ori_states)
  sec_sys_controller/1(Sec_inputs) -> Sum1/2, Observer/1(Sec_input)
  Observer/1(Sec_Obv_States) -> sec_sys_controller/2(Sec_Obv_States)
  F-16/2(V_wind) -> V_wind/1
  Observer/2(Pri_Obv_States) -> sec_sys_controller/1(Pri_Obv_States), pri_sys_controller/1(Pri_Obv_States)
  Sum1/1 -> F-16/2(u1)
  u2/1 -> F-16/1(u2)
  F-16/3(W_wind) -> W_wind/1
  pri_sys_controller/1(Pri_inputs) -> Sum1/1

== system AirRefueling_Platform_Varyingmass/Hose-drogue system/DRdynamics/Hose-Drogue1/Atmosphere Data ==
  height : Inport
  1-D Lookup Table : Lookup_n-D  NumberOfTableDimensions=1  BreakpointsForDimension1=[0,1000,2000,3000,4000,5000,6000,7000,8000,9000,10000]  Table=[1.789e-05,1.749e-05,1.717e-05,1.684e-05,1.652e-05,1.619e-05,1.586e-05,1.552e-05,1.517e-05,1.482e-05,1.447e-05]  RndMeth=Simplest
  COESA Atmosphere Model : aerolibatmos2/COESA Atmosphere Model  units=Metric (MKS)  spec=MIL-STD-210C  model=Profile  profile_var=High temperature  profile_percent=1%  profile_alt=5 km (16404 ft)  envelope_var=High temperature  envelope_percent=1%  action=Warning
  Terminator : Terminator
  Terminator1 : Terminator
  Terminator2 : Terminator
  densitiy : Outport
  viscosity : Outport  Port=2
  wires:
  COESA Atmosphere Model/4 -> densitiy/1
  height/1 -> 1-D Lookup Table/1, COESA Atmosphere Model/1
  COESA Atmosphere Model/1 -> Terminator/1
  COESA Atmosphere Model/2 -> Terminator1/1
  COESA Atmosphere Model/3 -> Terminator2/1
  1-D Lookup Table/1 -> viscosity/1

== system AirRefueling_Platform_Varyingmass/Hose-drogue system/DRdynamics/Hose-Drogue1/Calculate the Acceleration of the Links1 ==
  note: 得到第一根杆子的拉力
  note: 计算出第一根杆子的外力
  Q : Inport
  Mdr : Inport  Port=2
  n : Inport  Port=3
  dn : Inport  Port=4
  link line density : Inport  Port=5
  l1 length : Inport  Port=6
  DD l1 length : Inport  Port=7
  "tanker acceleration " : Inport  Port=8
  IC : InitialCondition  Value=0
  MATLAB Function : MATLAB Function  TreatAsAtomicUnit=on
  MATLAB Function2 : MATLAB Function  TreatAsAtomicUnit=on
  MATLAB Function3 : MATLAB Function  TreatAsAtomicUnit=on
  MATLAB Function4 : MATLAB Function  TreatAsAtomicUnit=on
  Product : Product
  a : Outport
  t : Outport  Port=2
  wires:
  n/1 -> MATLAB Function4/1(n), MATLAB Function3/3(n), MATLAB Function/1(n)
  Product/1 -> MATLAB Function3/4(m1), MATLAB Function4/4(m1), MATLAB Function/2(m1)  "l1 mass"
  Q/1 -> MATLAB Function4/3(Q), MATLAB Function3/2(Q)
  DD l1 length/1 -> MATLAB Function4/6(ddl1)
  "tanker acceleration "/1 -> MATLAB Function4/7(a0)
  dn/1 -> MATLAB Function4/2(dn)
  l1 length/1 -> MATLAB Function4/5(l1), Product/2
  link line density/1 -> Product/1
  MATLAB Function/1(T) -> MATLAB Function2/1(T)
  MATLAB Function4/1(q) -> MATLAB Function2/2(q)
  MATLAB Function2/2(t) -> IC/1
  Mdr/1 -> MATLAB Function3/5(Mdr)
  MATLAB Function3/1(a) -> a/1
  MATLAB Function2/1(t0) -> t/1
  IC/1 -> MATLAB Function3/1(t)

== system AirRefueling_Platform_Varyingmass/Hose-drogue system/DRdynamics/Hose-Drogue1/Calculate the External Force of the Links ==
  note: 计算雷诺数以及相应的摩擦系数Cf和压差系数Cd
  vr : Inport
  n : Inport  Port=2
  l1 : Inport  Port=3
  link radius : Inport  Port=4
  link line density : Inport  Port=5
  density : Inport  Port=6
  viscosity : Inport  Port=7
  p : Inport  Port=8
  Fb : Inport  Port=9
  Drogue Coeffecint : Constant  Value=Cdr_
  Drogue Mass : Constant  Value=Mdr
  Drogue Radius : Constant  Value=Rdr
  MATLAB Function : MATLAB Function  TreatAsAtomicUnit=on
  MATLAB Function1 : MATLAB Function  TreatAsAtomicUnit=on
  Scope{,1..9} (10 alike) : Scope
  Q : Outport
  Mdr : Outport  Port=2
  wires:
  MATLAB Function/1(Ref) -> Scope/1
  MATLAB Function/3(Red) -> Scope2/1
  MATLAB Function1/1(Q) -> Q/1
  vr/1 -> MATLAB Function/1(vr), MATLAB Function1/1(vr)
  n/1 -> MATLAB Function1/2(n), MATLAB Function/2(n)
  link radius/1 -> MATLAB Function/3(radius), MATLAB Function1/7(radius)
  viscosity/1 -> MATLAB Function/4(viscosity)
  density/1 -> MATLAB Function1/6(density)
  Drogue Radius/1 -> MATLAB Function1/8(Rdr)
  Drogue Coeffecint/1 -> MATLAB Function1/9(Cdr)
  Drogue Mass/1 -> Mdr/1, MATLAB Function1/10(Mdr)
  link line density/1 -> MATLAB Function1/11(rou)
  MATLAB Function1/2(Df_mid) -> Scope1/1
  MATLAB Function1/3(Dd_mid) -> Scope3/1
  MATLAB Function1/4(Df) -> Scope4/1
  MATLAB Function1/5(Dd) -> Scope5/1
  MATLAB Function1/6(D) -> Scope6/1
  MATLAB Function1/7(Ddr) -> Scope7/1
  MATLAB Function/2(Cf) -> MATLAB Function1/3(Cf)
  MATLAB Function/4(Cd) -> MATLAB Function1/4(Cd)
  p/1 -> MATLAB Function1/12(p)
  l1/1 -> MATLAB Function1/5(l1)
  Fb/1 -> MATLAB Function1/13(Fb)
  MATLAB Function1/8(fen_norm) -> Scope8/1
  MATLAB Function1/9(fen) -> Scope9/1

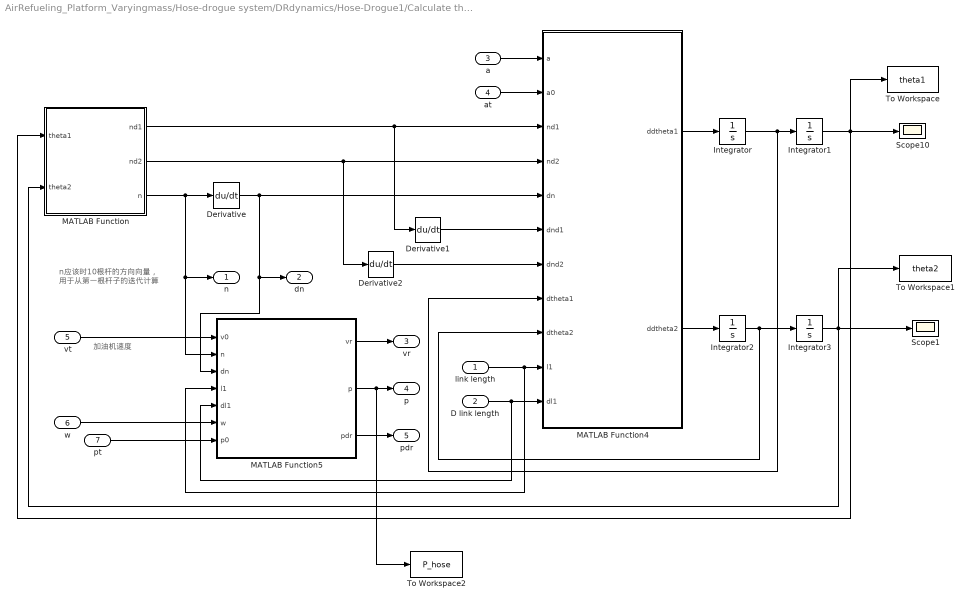
== system AirRefueling_Platform_Varyingmass/Hose-drogue system/DRdynamics/Hose-Drogue1/Calculate the Orientation of the Links1 ==
  note: n应该时10根杆的方向向量，
      | 用于从第一根杆子的迭代计算
  note: 加油机速度
  link length : Inport
  D link length : Inport  Port=2
  a : Inport  Port=3
  at : Inport  Port=4
  vt : Inport  Port=5
  w : Inport  Port=6
  pt : Inport  Port=7
  Derivative : Derivative
  Derivative1 : Derivative
  Derivative2 : Derivative
  Integrator : Integrator  InitialCondition=dtheta10
  Integrator1 : Integrator  InitialCondition=theta10
  Integrator2 : Integrator  InitialCondition=dtheta20
  Integrator3 : Integrator  InitialCondition=theta20
  MATLAB Function : MATLAB Function  TreatAsAtomicUnit=on
  MATLAB Function4 : MATLAB Function  TreatAsAtomicUnit=on
  MATLAB Function5 : MATLAB Function  TreatAsAtomicUnit=on
  Scope1 : Scope
  Scope10 : Scope
  To Workspace : ToWorkspace  VariableName=theta1  SampleTime=-1
      settings: Save2DSignal=2-D array (concatenate along first dimension)
  To Workspace1 : ToWorkspace  VariableName=theta2  SampleTime=-1
      settings: Save2DSignal=2-D array (concatenate along first dimension)
  To Workspace2 : ToWorkspace  VariableName=P_hose  SampleTime=-1
  n : Outport
  dn : Outport  Port=2
  vr : Outport  Port=3
  p : Outport  Port=4
  pdr : Outport  Port=5
  wires:
  Integrator1/1 -> To Workspace/1, MATLAB Function/1(theta1), Scope10/1
  Integrator3/1 -> To Workspace1/1, MATLAB Function/2(theta2), Scope1/1
  MATLAB Function/3(n) -> MATLAB Function5/2(n), n/1, Derivative/1
  Integrator/1 -> MATLAB Function4/8(dtheta1), Integrator1/1
  Integrator2/1 -> MATLAB Function4/9(dtheta2), Integrator3/1
  Derivative1/1 -> MATLAB Function4/6(dnd1)
  Derivative2/1 -> MATLAB Function4/7(dnd2)
  MATLAB Function4/2(ddtheta2) -> Integrator2/1
  link length/1 -> MATLAB Function4/10(l1), MATLAB Function5/4(l1)
  D link length/1 -> MATLAB Function5/5(dl1), MATLAB Function4/11(dl1)
  a/1 -> MATLAB Function4/1(a)
  at/1 -> MATLAB Function4/2(a0)
  vt/1 -> MATLAB Function5/1(v0)
  w/1 -> MATLAB Function5/6(w)
  MATLAB Function5/1(vr) -> vr/1
  pt/1 -> MATLAB Function5/7(p0)
  MATLAB Function/1(nd1) -> Derivative1/1, MATLAB Function4/3(nd1)
  MATLAB Function/2(nd2) -> Derivative2/1, MATLAB Function4/4(nd2)
  Derivative/1 -> MATLAB Function5/3(dn), dn/1, MATLAB Function4/5(dn)
  MATLAB Function5/3(pdr) -> pdr/1
  MATLAB Function5/2(p) -> To Workspace2/1, p/1
  MATLAB Function4/1(ddtheta1) -> Integrator/1

== system AirRefueling_Platform_Varyingmass/Receiver system/F16 Nonlinear Model/Variable Mass Model/Adding Wind Disturbance1 ==
  Speed of Sound : Inport
  Air Density : Inport  Port=2
  Wind Velocity : Inport  Port=3  PortDimensions=3
  Wind Angular Rates : Inport  Port=4  PortDimensions=3
  Vb : Inport  Port=5  PortDimensions=3
  p,q,r : Inport  Port=6  PortDimensions=3
  Display : Display
  Dynamic Pressure : aerolibasang/Dynamic Pressure
  "Incidence, Sideslip & Airspeed" : aerolibasang/Incidence, Sideslip, & Airspeed
  Mach Number : aerolibasang/Mach Number
  Mux : Mux  Inputs=2
  Sum : Sum  Inputs=|+-  InputSameDT=on  SaturateOnIntegerOverflow=on  OutDataTypeStr=Inherit: Same as first input
  Sum1 : Sum  Inputs=|++  InputSameDT=on  SaturateOnIntegerOverflow=on  OutDataTypeStr=Inherit: Same as first input
  qbar : Outport  InitialOutput=0
  "p,q,r " : Outport  Port=2
  V : Outport  Port=3
  Mach : Outport  Port=4
  Incid : Outport  Port=5
  wires:
  "Incidence, Sideslip & Airspeed"/3 -> V/1
  Dynamic Pressure/1 -> qbar/1
  Air Density/1 -> Dynamic Pressure/2
  Mach Number/1 -> Mach/1
  Sum/1 -> Dynamic Pressure/1, Mach Number/1, "Incidence, Sideslip & Airspeed"/1
  Vb/1 -> Display/1, Sum/1
  Speed of Sound/1 -> Mach Number/2
  Wind Velocity/1 -> Sum/2
  "Incidence, Sideslip & Airspeed"/2 -> Mux/2  "Beta"
  Mux/1 -> Incid/1
  "Incidence, Sideslip & Airspeed"/1 -> Mux/1  "Alpha"
  p,q,r/1 -> Sum1/1
  Wind Angular Rates/1 -> Sum1/2
  Sum1/1 -> "p,q,r "/1

== system AirRefueling_Platform_Varyingmass/Receiver system/F16 Nonlinear Model/Variable Mass Model/Aerodynamic Coefficients1 ==
  Actuators : Inport
  Incid : Inport  Port=2
  Mach : Inport  Port=3
  V : Inport  Port=4
  p,q,r : Inport  Port=5
  qbar/ps : Inport  Port=6
  Angle Conversion : aerolibconvert2/Angle Conversion  IU=rad  OU=deg
  Display : Display
  Interpreted MATLAB Function : MATLABFcn  MATLABFcn=F16Coef1  OutputDimensions=6
  Leading Edge Flap : Subsystem
  Mux : Mux  Inputs=6
  Terminator2 : Terminator
  alpha : Selector  InputPortWidth=2  IndexOptions=Index vector (dialog)  Indices=1  OutputSizes=1
  flag : Constant  Value=fi_flag
  Coeff : Outport  InitialOutput=0
  wires:
  Angle Conversion/1 -> alpha/1, Mux/2
  Incid/1 -> Angle Conversion/1
  qbar/ps/1 -> Leading Edge Flap/2(qbar/ps)
  alpha/1 -> Leading Edge Flap/1(alpha)
  V/1 -> Display/1, Mux/1
  p,q,r/1 -> Mux/3
  Actuators/1 -> Mux/4
  flag/1 -> Mux/5
  Mach/1 -> Terminator2/1
  Interpreted MATLAB Function/1 -> Coeff/1
  Mux/1 -> Interpreted MATLAB Function/1
  Leading Edge Flap/1(delta_lef (deg)) -> Mux/6

== system AirRefueling_Platform_Varyingmass/Receiver system/F16 Nonlinear Model/Variable Mass Model/Environment Models ==
  Xe : Inport  PortDimensions=3
  DCM : Inport  Port=2
  COESA Atmosphere Model : aerolibatmos2/COESA Atmosphere Model  units=English (Velocity in ft/s)  spec=1976 COESA-extended U.S. Standard Atmosphere  model=Profile  profile_var=High temperature  profile_percent=10%  profile_alt=5 km (16404 ft)  envelope_var=High temperature  envelope_percent=1%  action=None
  Gravity in Earth Axes : Gain  Gain=mass  SaturateOnIntegerOverflow=on  OutDataTypeStr=Inherit: Same as input  ParamDataTypeStr=Inherit: Same as input
  Height : Selector  InputPortWidth=3  IndexOptions=Index vector (dialog)  Indices=[3]  OutputSizes=1
  Inertial to Body : Product  Multiplication=Matrix(*)  InputSameDT=on  SaturateOnIntegerOverflow=on  OutDataTypeStr=Inherit: Same as first input
  Latitude : Constant  Value=0
  Mux : Mux  Inputs=3
  Product6 : Product  Inputs=**  InputSameDT=on  SaturateOnIntegerOverflow=on  OutDataTypeStr=Inherit: Same as first input
  Reshape : Reshape
  Terminator : Terminator
  "WGS84 Gravity Model " : aerolibobsolete/WGS84 Gravity Model   model=WGS84 Taylor Series  units=English  no_atmos=on  precessing=on  jd_loc=off  month=October  day=10  year=2004  no_centrifugal=on  action=None
  r2d5 : Gain  Gain=1715  SaturateOnIntegerOverflow=on  OutDataTypeStr=Inherit: Same as input  ParamDataTypeStr=Inherit: Same as input
  z-->h : Abs
  Fg : Outport  InitialOutput=0  VectorParamsAs1DForOutWhenUnconnected=off
  Speed of Sound : Outport  Port=2  InitialOutput=0  VectorParamsAs1DForOutWhenUnconnected=off
  Air Density : Outport  Port=3  InitialOutput=0  VectorParamsAs1DForOutWhenUnconnected=off
  PS : Outport  Port=4  VectorParamsAs1DForOutWhenUnconnected=off
  wires:
  Reshape/1 -> Inertial to Body/2
  Mux/1 -> "WGS84 Gravity Model "/1
  z-->h/1 -> Mux/3, COESA Atmosphere Model/1
  COESA Atmosphere Model/2 -> Speed of Sound/1
  COESA Atmosphere Model/3 -> Terminator/1
  Height/1 -> z-->h/1
  Xe/1 -> Height/1
  Latitude/1 -> Mux/2, Mux/1
  "WGS84 Gravity Model "/1 -> Gravity in Earth Axes/1
  Gravity in Earth Axes/1 -> Reshape/1
  DCM/1 -> Inertial to Body/1
  Inertial to Body/1 -> Fg/1
  COESA Atmosphere Model/4 -> Product6/2, Air Density/1
  COESA Atmosphere Model/1 -> r2d5/1
  Product6/1 -> PS/1
  r2d5/1 -> Product6/1

== system AirRefueling_Platform_Varyingmass/Receiver system/F16 Nonlinear Model/Variable Mass Model/Forces and Moments1 ==
  Coeff : Inport
  Thrust : Inport  Port=2
  qbar : Inport  Port=3
  "Aerodynamic Forces and Moments " : aerolibadyn/Aerodynamic Forces and Moments   inputAxes=Body  outputForceAxes=Body  outputMomentAxes=Body  S=S_ref  b=b_ref  cbar=d_ref
  Center of Gravity : Constant  Value=[-0 0 0]
  Center of Pressure : Constant  Value=[-0 0 0]
  Sum : Sum  Inputs=++|  InputSameDT=on  SaturateOnIntegerOverflow=on  OutDataTypeStr=Inherit: Same as first input
  X,Y,Z : Outport  InitialOutput=0
  LMN : Outport  Port=2  InitialOutput=0
  wires:
  Center of Pressure/1 -> "Aerodynamic Forces and Moments "/4
  Center of Gravity/1 -> "Aerodynamic Forces and Moments "/3
  "Aerodynamic Forces and Moments "/1 -> Sum/2
  "Aerodynamic Forces and Moments "/2 -> LMN/1
  Sum/1 -> X,Y,Z/1
  Thrust/1 -> Sum/1
  qbar/1 -> "Aerodynamic Forces and Moments "/2
  Coeff/1 -> "Aerodynamic Forces and Moments "/1

== system AirRefueling_Platform_Varyingmass/Receiver system/F16 Nonlinear Model/Variable Mass Model/actuator1 ==
  u : Inport
  Aileron Actuator : Subsystem
  Demux : Demux
  Elevator Actuator : Subsystem
  Mux1 : Mux  Inputs=3
  Mux2 : Mux  Inputs=3
  Rudder Actuator : Subsystem
  Thrust Model : Subsystem
  Ty : Constant  Value=0
  Tz : Constant  Value=0
  Ang : Outport
  T : Outport  Port=2
  wires:
  u/1 -> Demux/1
  Mux2/1 -> Ang/1
  Thrust Model/1(T) -> Mux1/1  "Tx"
  Ty/1 -> Mux1/2
  Tz/1 -> Mux1/3
  Mux1/1 -> T/1
  Demux/1 -> Thrust Model/1(delta_t)
  Elevator Actuator/1(el) -> Mux2/1  "el"
  Aileron Actuator/1(ail) -> Mux2/2  "ail"
  Rudder Actuator/1(rud) -> Mux2/3  "rud"
  Demux/2 -> Elevator Actuator/1(delta_e)
  Demux/3 -> Aileron Actuator/1(delta_a)
  Demux/4 -> Rudder Actuator/1(delta_r)

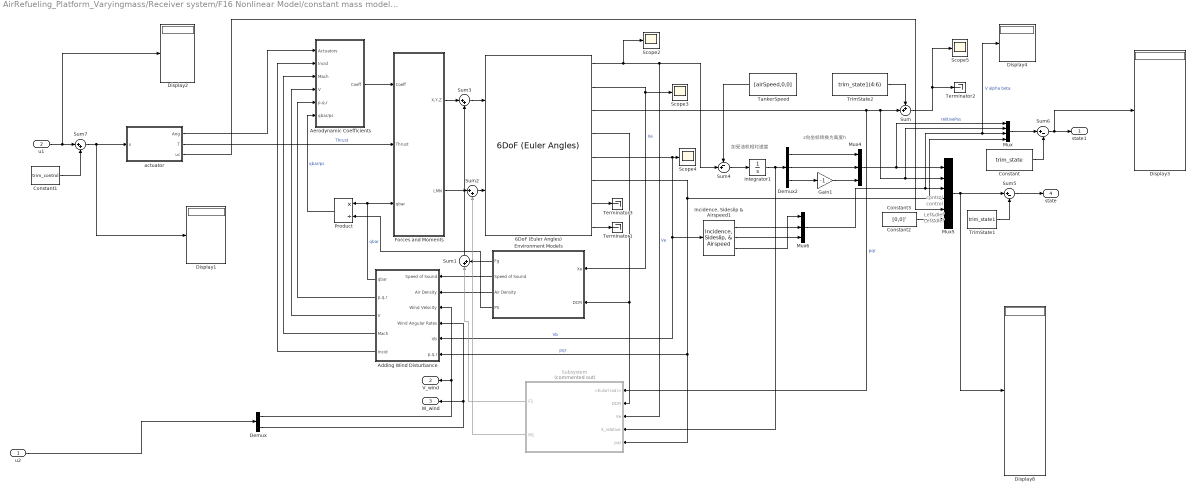
== system AirRefueling_Platform_Varyingmass/Receiver system/F16 Nonlinear Model/constant mass model/F-16 ==
  note: 加受油机相对速度
  note: z向坐标转换为高度h
  note: Lef&dlef
  note: control
  note: control
  note: Lef&dlef
  u2 : Inport
  u1 : Inport  Port=2
  6DoF (Euler Angles) : aerolibobsolete/6DoF (Euler Angles)  units=English (Velocity in ft/s)  mtype=Fixed  rep=Euler Angles  xme_0=xyz_0  Vm_0=uvw_0  eul_0=Euler_0  pm_0=pqr  mass_0=mass  mass_e=0.5  mass_f=2.0  inertia=Inertia  inertia_e=eye(3)  inertia_f=2*eye(3)  k_quat=1.0
  Adding Wind Disturbance : Subsystem
  Aerodynamic Coefficients : Subsystem
  Constant : Constant  Value=trim_state
  Constant1 : Constant  Value=trim_control
  Constant2 : Constant  Value=[0,0]'
  Constant3 : Constant  Value=[0,0]'
  Demux : Demux  Outputs=2
  Demux2 : Demux  Outputs=3
  Display{1..4,8} (5 alike) : Display
  Environment Models : Subsystem
  Forces and Moments : Subsystem
  Gain1 : Gain  Gain=-1
  "Incidence, Sideslip & Airspeed1" : aerolibasang/Incidence, Sideslip, & Airspeed
  Integrator1 : Integrator
  Mux : Mux
  Mux4 : Mux  Inputs=3
  Mux5 : Mux  Inputs=6
  Mux6 : Mux  Inputs=3
  Product : Product  Inputs=*/  InputSameDT=on  SaturateOnIntegerOverflow=on  OutDataTypeStr=Inherit: Same as first input
  Scope{2..5} (4 alike) : Scope
  Subsystem : Subsystem  Commented=on
  Sum : Sum  Inputs=++|
  Sum1 : Sum  Inputs=|++  InputSameDT=on  SaturateOnIntegerOverflow=on  OutDataTypeStr=Inherit: Same as first input
  Sum2 : Sum  Inputs=|++  InputSameDT=on  SaturateOnIntegerOverflow=on  OutDataTypeStr=Inherit: Same as first input
  Sum3 : Sum  Inputs=|++  InputSameDT=on  SaturateOnIntegerOverflow=on  OutDataTypeStr=Inherit: Same as first input
  Sum4 : Sum  Inputs=-+|
  Sum5 : Sum  Inputs=|+-
  Sum6 : Sum  Inputs=|+-
  Sum7 : Sum  Inputs=|++
  TankerSpeed : Constant  Value=[airSpeed,0,0]
  Terminator1 : Terminator
  Terminator2 : Terminator
  Terminator3 : Terminator
  TrimState1 : Constant  Value=trim_state1
  TrimState2 : Constant  Value=trim_state1(4:6)
  actuator : Subsystem
  state1 : Outport
  V_wind : Outport  Port=2  VectorParamsAs1DForOutWhenUnconnected=off
  W_wind : Outport  Port=3  VectorParamsAs1DForOutWhenUnconnected=off
  state : Outport  Port=4
  wires:
  Sum3/1 -> 6DoF (Euler Angles)/1
  Sum/1 -> Terminator2/1, Scope5/1
  6DoF (Euler Angles)/1 -> Scope2/1, Sum4/2, Subsystem/3(Ve)  "Ve"
  actuator/2(T) -> Forces and Moments/2(Thrust)  "Thrust"
  Adding Wind Disturbance/1(qbar) -> Forces and Moments/3(qbar), Product/1  "qbar"
  "Incidence, Sideslip & Airspeed1"/1 -> Mux6/2
  u1/1 -> Display2/1, Sum7/1
  Constant3/1 -> Mux5/6
  Sum1/1 -> Sum3/2
  Forces and Moments/1(X,Y,Z) -> Sum3/1
  Mux6/1 -> Display4/1, Mux/3, Mux5/3  "V alpha beta"
  Forces and Moments/2(LMN) -> Sum2/1
  u2/1 -> Demux/1
  Constant/1 -> Sum6/2
  Environment Models/3(Air Density) -> Adding Wind Disturbance/2(Air Density)
  "Incidence, Sideslip & Airspeed1"/2 -> Mux6/3
  Mux/1 -> Sum6/1
  Sum6/1 -> state1/1, Display3/1
  Mux4/1 -> Mux/1, Mux5/1  "relitivePos"
  Adding Wind Disturbance/2("p,q,r ") -> Aerodynamic Coefficients/5(p,q,r)
  6DoF (Euler Angles)/8 -> Terminator1/1
  6DoF (Euler Angles)/5 -> Scope4/1, Adding Wind Disturbance/5(Vb), "Incidence, Sideslip & Airspeed1"/1  "Vb"
  Environment Models/2(Speed of Sound) -> Adding Wind Disturbance/1(Speed of Sound)
  Aerodynamic Coefficients/1(Coeff) -> Forces and Moments/1(Coeff)
  Adding Wind Disturbance/5(Incid) -> Aerodynamic Coefficients/2(Incid)
  Adding Wind Disturbance/3(V) -> Aerodynamic Coefficients/4(V)
  Sum2/1 -> 6DoF (Euler Angles)/2
  6DoF (Euler Angles)/7 -> Terminator3/1
  Mux5/1 -> Sum5/1, Display8/1
  actuator/1(Ang) -> Aerodynamic Coefficients/1(Actuators)
  Constant1/1 -> Sum7/2
  Sum7/1 -> Display1/1, actuator/1(u)
  "Incidence, Sideslip & Airspeed1"/3 -> Mux6/1
  Demux2/3 -> Gain1/1
  Adding Wind Disturbance/4(Mach) -> Aerodynamic Coefficients/3(Mach)
  Environment Models/1(Fg) -> Sum1/2
  TankerSpeed/1 -> Sum4/1
  6DoF (Euler Angles)/2 -> Scope3/1, Environment Models/1(Xe)  "Xe"
  Sum4/1 -> Integrator1/1
  Gain1/1 -> Mux4/3
  Demux2/2 -> Mux4/2
  Product/1 -> Aerodynamic Coefficients/6(qbar/ps)  "qbar/ps"
  Demux2/1 -> Mux4/1
  Environment Models/4(PS) -> Product/2
  TrimState2/1 -> Sum/1
  Demux/1 -> V_wind/1, Adding Wind Disturbance/3(Wind Velocity)
  Demux/2 -> W_wind/1, Adding Wind Disturbance/4(Wind Angular Rates)
  Subsystem/2(M1) -> Sum2/2
  Integrator1/1 -> Subsystem/4(X_relative), Demux2/1
  Subsystem/1(F1) -> Sum1/1
  6DoF (Euler Angles)/4 -> Subsystem/2(DCM), Environment Models/2(DCM)
  actuator/3(uc) -> Mux5/5
  6DoF (Euler Angles)/6 -> Subsystem/5(pqr), Adding Wind Disturbance/6(p,q,r), Mux/4, Mux5/4  "pqr"
  6DoF (Euler Angles)/3 -> Subsystem/1(<Eular(rad)>), Mux/2, Mux5/2, Sum/2  "pqr"
  Sum5/1 -> state/1
  TrimState1/1 -> Sum5/2

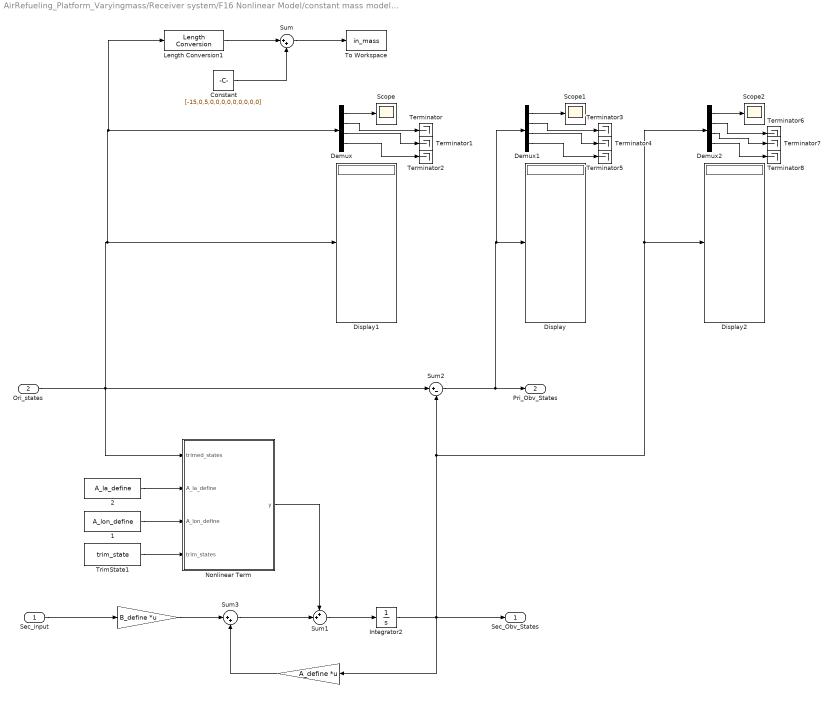
== system AirRefueling_Platform_Varyingmass/Receiver system/F16 Nonlinear Model/constant mass model/Observer ==
  Sec_input : Inport
  Ori_states : Inport  Port=2
  " " : Gain  Gain=A_define  Multiplication=Matrix(K*u) (u vector)
  "  " : Gain  Gain=B_define  Multiplication=Matrix(K*u) (u vector)
  " 1" : Constant  Value=A_lon_define
  " 2" : Constant  Value=A_la_define
  Constant : Constant  Value=[-15,0,5,0,0,0,0,0,0,0,0,0]
  Demux : Demux
  Demux1 : Demux
  Demux2 : Demux
  Display : Display
  Display1 : Display
  Display2 : Display
  Integrator2 : Integrator
  Length Conversion1 : aerolibconvert2/Length Conversion  IU=ft  OU=m
  Nonlinear Term : MATLAB Function  TreatAsAtomicUnit=on
  Scope : Scope
  Scope1 : Scope
  Scope2 : Scope
  Sum : Sum  Inputs=|++
  Sum1 : Sum  Inputs=++|
  Sum2 : Sum  Inputs=|+-
  Sum3 : Sum  Inputs=|++
  Terminator{,1..8} (9 alike) : Terminator
  To Workspace : ToWorkspace  VariableName=in_mass  SaveFormat=Structure With Time  SampleTime=-1
  TrimState1 : Constant  Value=trim_state
  Sec_Obv_States : Outport  VectorParamsAs1DForOutWhenUnconnected=off
  Pri_Obv_States : Outport  Port=2  VectorParamsAs1DForOutWhenUnconnected=off
  wires:
  Sec_input/1 -> "  "/1
  "  "/1 -> Sum3/1
  " "/1 -> Sum3/2
  Sum3/1 -> Sum1/2
  Sum1/1 -> Integrator2/1
  Integrator2/1 -> Sec_Obv_States/1, " "/1, Demux2/1, Display2/1, Sum2/2
  Sum2/1 -> Demux1/1, Display/1, Pri_Obv_States/1
  " 1"/1 -> Nonlinear Term/3(A_lon_define)
  " 2"/1 -> Nonlinear Term/2(A_la_define)
  Demux/1 -> Scope/1
  Demux1/1 -> Scope1/1
  Demux2/1 -> Scope2/1
  Nonlinear Term/1(y) -> Sum1/1
  TrimState1/1 -> Nonlinear Term/4(trim_states)
  Ori_states/1 -> Sum2/1, Length Conversion1/1, Demux/1, Display1/1, Nonlinear Term/1(trimed_states)
  Constant/1 -> Sum/2
  Sum/1 -> To Workspace/1
  Length Conversion1/1 -> Sum/1
  Demux/4 -> Terminator2/1
  Demux/3 -> Terminator1/1
  Demux/2 -> Terminator/1
  Demux1/4 -> Terminator5/1
  Demux1/3 -> Terminator4/1
  Demux1/2 -> Terminator3/1
  Demux2/4 -> Terminator8/1
  Demux2/2 -> Terminator6/1
  Demux2/3 -> Terminator7/1

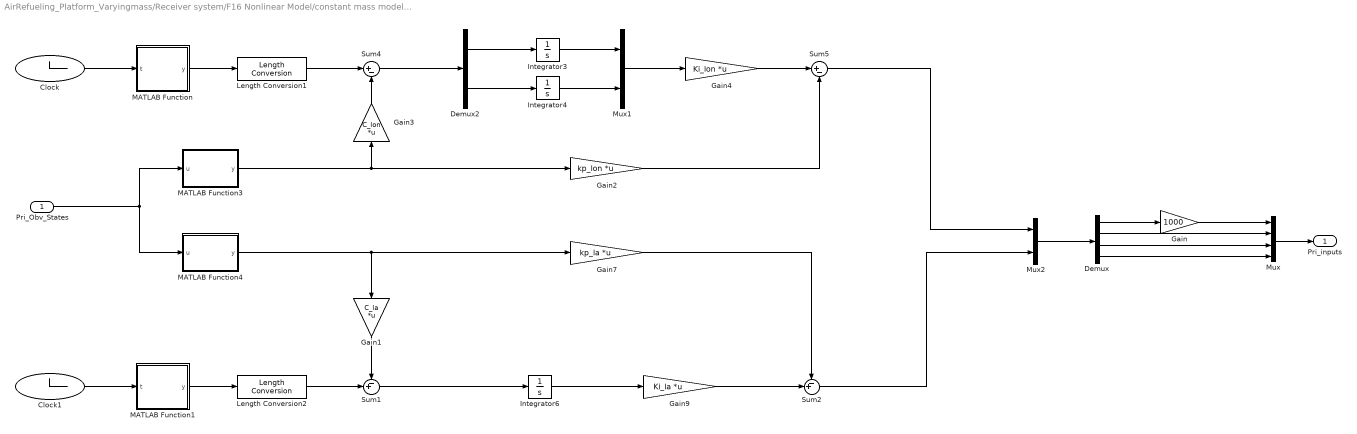
== system AirRefueling_Platform_Varyingmass/Receiver system/F16 Nonlinear Model/constant mass model/pri_sys_controller ==
  Pri_Obv_States : Inport
  Clock : Clock
      settings: Decimation=50
  Clock1 : Clock
      settings: Decimation=50
  Demux : Demux
  Demux2 : Demux  Outputs=2
  Gain : Gain  Gain=1000
  Gain1 : Gain  Gain=C_la  Multiplication=Matrix(K*u) (u vector)
  Gain2 : Gain  Gain=kp_lon  Multiplication=Matrix(K*u) (u vector)
  Gain3 : Gain  Gain=C_lon  Multiplication=Matrix(K*u) (u vector)
  Gain4 : Gain  Gain=Ki_lon  Multiplication=Matrix(K*u) (u vector)
  Gain7 : Gain  Gain=kp_la  Multiplication=Matrix(K*u) (u vector)
  Gain9 : Gain  Gain=Ki_la  Multiplication=Matrix(K*u) (u vector)
  Integrator3 : Integrator
  Integrator4 : Integrator
  Integrator6 : Integrator
  Length Conversion1 : aerolibconvert2/Length Conversion  IU=m  OU=ft
  Length Conversion2 : aerolibconvert2/Length Conversion  IU=m  OU=ft
  MATLAB Function : MATLAB Function  TreatAsAtomicUnit=on
  MATLAB Function1 : MATLAB Function  TreatAsAtomicUnit=on
  MATLAB Function3 : MATLAB Function  TreatAsAtomicUnit=on
  MATLAB Function4 : MATLAB Function  TreatAsAtomicUnit=on
  Mux : Mux
  Mux1 : Mux  Inputs=2
  Mux2 : Mux  Inputs=2
  Sum1 : Sum  Inputs=-+|
  Sum2 : Sum  Inputs=-+|
  Sum4 : Sum  Inputs=|+-
  Sum5 : Sum  Inputs=|+-
  Pri_inputs : Outport  VectorParamsAs1DForOutWhenUnconnected=off
  wires:
  Pri_Obv_States/1 -> MATLAB Function3/1(u), MATLAB Function4/1(u)
  Gain2/1 -> Sum5/2
  MATLAB Function/1(y) -> Length Conversion1/1
  Sum4/1 -> Demux2/1
  Demux2/2 -> Integrator4/1
  Integrator4/1 -> Mux1/2
  Integrator3/1 -> Mux1/1
  Mux1/1 -> Gain4/1
  Gain3/1 -> Sum4/2
  Gain4/1 -> Sum5/1
  Clock/1 -> MATLAB Function/1(t)
  Length Conversion1/1 -> Sum4/1
  Demux/2 -> Mux/2
  Demux/3 -> Mux/3
  Demux/4 -> Mux/4
  Demux/1 -> Gain/1
  Gain/1 -> Mux/1
  Mux/1 -> Pri_inputs/1
  MATLAB Function1/1(y) -> Length Conversion2/1
  Sum1/1 -> Integrator6/1
  Integrator6/1 -> Gain9/1
  Clock1/1 -> MATLAB Function1/1(t)
  MATLAB Function3/1(y) -> Gain2/1, Gain3/1
  MATLAB Function4/1(y) -> Gain7/1, Gain1/1
  Length Conversion2/1 -> Sum1/2
  Gain1/1 -> Sum1/1
  Gain9/1 -> Sum2/2
  Gain7/1 -> Sum2/1
  Sum5/1 -> Mux2/1
  Sum2/1 -> Mux2/2
  Demux2/1 -> Integrator3/1
  Mux2/1 -> Demux/1
